simulink model "RDataGeneration"  (R2017b)
settings: Solver=ode5  StartTime=0.0  StopTime=85500  FixedStep=0.0025  RelTol=1e-3  AbsTol=1e-6
libraries: DABLib x6
settings Model: Creator=davidlaredorazo  LastModifiedBy=davidlaredorazo
settings DataIOCC: SaveFormat=Array  SignalLoggingSaveFormat=ModelDataLogs
settings OptimizationCC: BlockReduction=off  BooleanDataType=off
settings DebuggingCC: SaveWithParameterizedLinksMsg=none  UnderspecifiedInitializationDetection=Classic  MergeDetectMultiDrivingBlocksExec=none  SignalResolutionControl=TryResolveAllWithWarning  MultiTaskDSMMsg=warning  MultiTaskCondExecSysMsg=none
settings HardwareCC: TargetUnknown=on
settings ModelReferenceCC: PropagateSignalLabelsOutOfModel=off
settings GRTTargetCC: TargetLangStandard=C89/C90 (ANSI)  CombineOutputUpdateFcns=off  GRTInterface=on

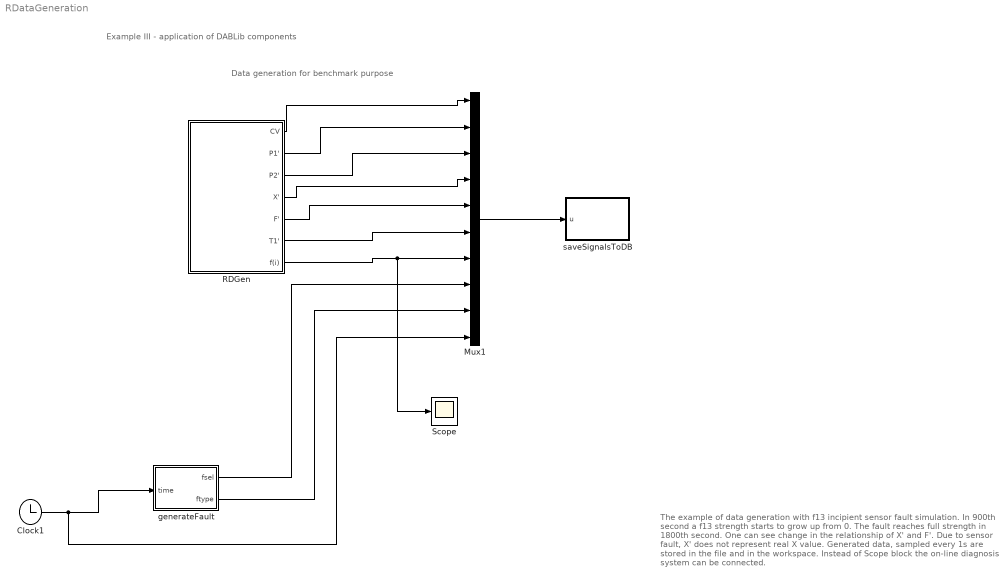
== system RDataGeneration ==
  note: Data generation for benchmark purpose
  note: Example III - application of DABLib components
  note: The example of data generation with f13 incipient sensor fault simulation.
      | In 900th second a f13 strength starts to grow up from 0.
      | The fault reaches full strength in 1800th second.
      | One can see change in the relationship of X' and F'.
      | Due to sensor fault, X' does not represent real X value.
      | Generated data, sampled every 1s are stored in the file and in the workspace.
      | Instead of Scope block the on-line diagnosis system can be connected.
  Clock1 : Clock
  Mux1 : Mux  Inputs=10
  RDGen : Subsystem
  Scope : Scope
  generateFault : MATLAB Function  TreatAsAtomicUnit=on
  saveSignalsToDB : MATLAB Function  TreatAsAtomicUnit=on
  wires:
  RDGen/1(CV) -> Mux1/1
  RDGen/3(P2') -> Mux1/3
  RDGen/4(X') -> Mux1/4
  RDGen/5(F') -> Mux1/5
  RDGen/6(T1') -> Mux1/6
  Clock1/1 -> Mux1/10, generateFault/1(time)
  generateFault/1(fsel) -> Mux1/8
  generateFault/2(ftype) -> Mux1/9
  RDGen/2(P1') -> Mux1/2
  RDGen/7(f(i)) -> Scope/1, Mux1/7
  Mux1/1 -> saveSignalsToDB/1(u)

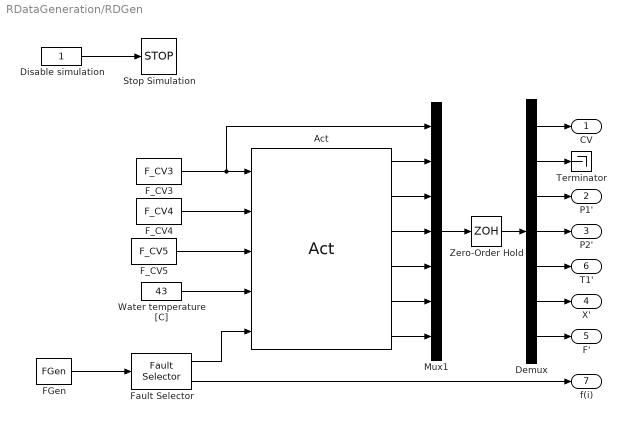
== system RDataGeneration/RDGen ==
  Act : DABLib/Act  Dist=off
  Demux : Demux  Outputs=7
  Disable simulation : Constant
  FGen : DABLib/FGen  From=FFrom  To=FTo  MFS=FMFS  FDT=FFDT  FSD=FSD
      link override Constant5: Value=1
      link override Ramp: start=1.0072  slope=1e+26
      link override Step: Time=1e+26
  F_CV3 : DABLib/DGen/F_CV3  A=0.25  f=0.01  c=0.5
  F_CV4 : DABLib/DGen/F_CV4  A=175000  f=0.1  c=3500000
  F_CV5 : DABLib/DGen/F_CV5  A=26000  f=1/pi  c=2600000
  Fault Selector : DABLib/DGen/Fault Selector
      link override Constant4: Value=10
  Mux1 : Mux  Inputs=7
  Stop Simulation : Stop
  Terminator : Terminator
  "Water temperature [C] " : Constant  Value=43
  Zero-Order Hold : ZeroOrderHold
  CV : Outport  InitialOutput=0
  P1' : Outport  Port=2  InitialOutput=0
  P2' : Outport  Port=3  InitialOutput=0
  X' : Outport  Port=4  InitialOutput=0
  F' : Outport  Port=5  InitialOutput=0
  T1' : Outport  Port=6  InitialOutput=0
  f(i) : Outport  Port=7  InitialOutput=0
  wires:
  Act/6 -> Mux1/7
  Zero-Order Hold/1 -> Demux/1
  Demux/1 -> CV/1
  Demux/4 -> P2'/1
  FGen/1 -> Fault Selector/1
  Act/2 -> Mux1/3
  Demux/2 -> Terminator/1
  Disable simulation/1 -> Stop Simulation/1
  Demux/3 -> P1'/1
  Demux/7 -> F'/1
  Act/3 -> Mux1/4
  Mux1/1 -> Zero-Order Hold/1
  F_CV5/1 -> Act/3
  Act/1 -> Mux1/2
  "Water temperature [C] "/1 -> Act/4
  Act/5 -> Mux1/6
  Act/4 -> Mux1/5
  Fault Selector/1 -> Act/5
  Demux/6 -> X'/1
  Demux/5 -> T1'/1
  Fault Selector/2 -> f(i)/1
  F_CV3/1 -> Mux1/1, Act/1
  F_CV4/1 -> Act/2

== matlab function RDataGeneration/generateFault ==
  data: time input; fsel output; ftype output
function [fsel, ftype] = GetRandomFault(time)

coder.extrinsic('RandomFaultGenerator');
DGenBlockAddress = 'RDataGeneration/RDGen';

fsel = 0;
ftype = 0;
[fsel, ftype] = RandomFaultGenerator(time, DGenBlockAddress);
%fprintf(2, "%f", fsel)

end

== matlab function RDataGeneration/saveSignalsToDB ==
  data: u input
function saveToDB(u)

coder.extrinsic('saveToDB');

saveToDB(u);

end
